simulink model "test_1"  (R2021a)
settings: Solver=ode8  StartTime=0.0  StopTime=6  FixedStep=ts  RelTol=1e-3
undefined symbols (not defined in the file or in its folder): Acid, Lead, ts
libraries: spsDiodeLib x14, spsMosfetLib x12, spsSeriesRLCBranchLib x10, spsCurrentMeasurementLib x8, simulink x7, spsBatteryLib x6, pid_lib x6, spsParallelRLCBranchLib x5, spsMeanLib x3, spsPWMGeneratorDCDCLib x2, spsOnDelayLib x2, spsVoltageMeasurementLib x2
settings Model: Creator=Aditya  LastModifiedBy=Aditya

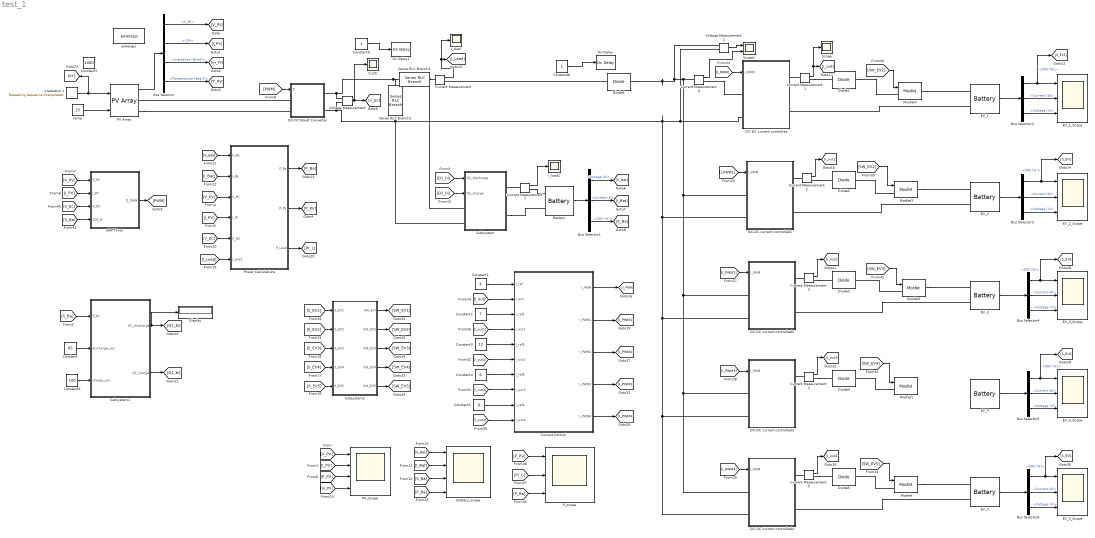
== system test_1 ==
  Battery : spsBatteryLib/Battery  BatType=Lead-Acid  ShowTempParam=off  ThermalPreset=no  ShowAgeParam=off  NomV=60  NomQ=150  SOC=65.01  Batt_Tr=0.1  PresetModel=on  MaxQ=156.25  MinV=45  FullV=65.3289  Dis_rate=30  R=0.004  Normal_OP=46.5417  expZone="[61.0855          0.5]"  current=[6.5 13 32.5]  Units=Time  Tci=20  NomT=20  T2=-30  MaxQ2=4.8  FullV2=7.1  Normal_OP2=5.655  expZone2="[6.58           1]"  Rca=0.6  ti=2000  Dp=0  Neq0=0  Tsim=1e6  Ta1=25  Qeol=5.4*0.9  Reol=0.013333*1.2  Char_age=[2.3478, 3]  Dis_age=[2.3478, 10]  N1=1500  N2=10500  N3=1000  N4=1400  Ta2=45  N5=950
  "Battery_scope " : Scope  NumInputPorts=4
  Bus Selector : BusSelector  OutputSignals=V_PV,I_PV,Irradiance (W/m2),Temperature (deg C)
  Bus Selector1 : BusSelector  OutputSignals=Voltage (V),Current (A),SOC (%)
  Bus Selector{2..6} (5 alike) : BusSelector  OutputSignals=SOC (%),Current (A),Voltage (V)
  Constant : Constant  Value=65
  Constant1 : Constant  Value=4
  Constant2 : Constant  Value=7
  Constant3 : Constant  Value=12
  Constant4 : Constant  Value=6
  Constant5 : Constant  Value=9
  Constant6 : Constant  Value=100
  Constant7 : Constant  Value=1000
  Constant8 : Constant
  Constant9 : Constant
  Current Control : Subsystem
  Current Measurement{,1..7} (8 alike) : spsCurrentMeasurementLib/Current Measurement  PhasorSimulation=off  OutputType=Complex  PSBequivalent=0
  DC-DC Boost Converter : Subsystem
  DC-DC current controlled : Subsystem
  DC-DC current controlled1 : Subsystem
  DC-DC current controlled2 : Subsystem
  DC-DC current controlled3 : Subsystem
  DC-DC current controlled4 : Subsystem
  Diode{1..6} (6 alike) : spsDiodeLib/Diode  Ron=0.001  Lon=0  Vf=0.8  IC=0  UseSnubber=0  Rs=500  Cs=250e-9  Measurements=off
  Display : Display
  EV_1 : spsBatteryLib/Battery  BatType=Lead-Acid  ShowTempParam=off  ThermalPreset=no  ShowAgeParam=off  NomV=48  NomQ=20  SOC=99.7  Batt_Tr=0.1  PresetModel=on  MaxQ=20.8333  MinV=36  FullV=52.2632  Dis_rate=4  R=0.024  Normal_OP=6.2056  expZone="[48.8684    0.0666667]"  current=[6.5 13 32.5]  Units=Time  Tci=20  NomT=20  T2=-30  MaxQ2=4.8  FullV2=7.1  Normal_OP2=5.655  expZone2="[6.58           1]"  Rca=0.6  ti=2000  Dp=0  Neq0=0  Tsim=1e6  Ta1=25  Qeol=5.4*0.9  Reol=0.013333*1.2  Char_age=[2.3478, 3]  Dis_age=[2.3478, 10]  N1=1500  N2=10500  N3=1000  N4=1400  Ta2=45  N5=950
  EV_1_Scope : Scope  NumInputPorts=3
  EV_2 : spsBatteryLib/Battery  BatType=Lead-Acid  ShowTempParam=off  ThermalPreset=no  ShowAgeParam=off  NomV=48  NomQ=30  SOC=99.8  Batt_Tr=0.1  PresetModel=on  MaxQ=31.25  MinV=36  FullV=52.2632  Dis_rate=6  R=0.016  Normal_OP=9.3083  expZone="[48.8684          0.1]"  current=[6.5 13 32.5]  Units=Time  Tci=20  NomT=20  T2=-30  MaxQ2=4.8  FullV2=7.1  Normal_OP2=5.655  expZone2="[6.58           1]"  Rca=0.6  ti=2000  Dp=0  Neq0=0  Tsim=1e6  Ta1=25  Qeol=5.4*0.9  Reol=0.013333*1.2  Char_age=[2.3478, 3]  Dis_age=[2.3478, 10]  N1=1500  N2=10500  N3=1000  N4=1400  Ta2=45  N5=950
  EV_2_Scope : Scope  NumInputPorts=3
  EV_3 : spsBatteryLib/Battery  BatType=Lead-Acid  ShowTempParam=off  ThermalPreset=no  ShowAgeParam=off  NomV=48  NomQ=50  SOC=99.9  Batt_Tr=0.1  PresetModel=on  MaxQ=52.0833  MinV=36  FullV=52.2632  Dis_rate=10  R=0.0096  Normal_OP=15.5139  expZone="[48.8684     0.166667]"  current=[6.5 13 32.5]  Units=Time  Tci=20  NomT=20  T2=-30  MaxQ2=4.8  FullV2=7.1  Normal_OP2=5.655  expZone2="[6.58           1]"  Rca=0.6  ti=2000  Dp=0  Neq0=0  Tsim=1e6  Ta1=25  Qeol=5.4*0.9  Reol=0.013333*1.2  Char_age=[2.3478, 3]  Dis_age=[2.3478, 10]  N1=1500  N2=10500  N3=1000  N4=1400  Ta2=45  N5=950
  EV_3_Scope : Scope  NumInputPorts=3
  EV_4 : spsBatteryLib/Battery  BatType=Lead-Acid  ShowTempParam=off  ThermalPreset=no  ShowAgeParam=off  NomV=48  NomQ=28  SOC=99.95  Batt_Tr=0.1  PresetModel=on  MaxQ=29.1667  MinV=36  FullV=52.2632  Dis_rate=5.6  R=0.017143  Normal_OP=8.6878  expZone="[48.8684    0.0933333]"  current=[6.5 13 32.5]  Units=Time  Tci=20  NomT=20  T2=-30  MaxQ2=4.8  FullV2=7.1  Normal_OP2=5.655  expZone2="[6.58           1]"  Rca=0.6  ti=2000  Dp=0  Neq0=0  Tsim=1e6  Ta1=25  Qeol=5.4*0.9  Reol=0.013333*1.2  Char_age=[2.3478, 3]  Dis_age=[2.3478, 10]  N1=1500  N2=10500  N3=1000  N4=1400  Ta2=45  N5=950
  EV_4_Scope : Scope  NumInputPorts=3
  EV_5 : spsBatteryLib/Battery  BatType=Lead-Acid  ShowTempParam=off  ThermalPreset=no  ShowAgeParam=off  NomV=48  NomQ=40  SOC=99.5  Batt_Tr=0.1  PresetModel=on  MaxQ=41.6667  MinV=36  FullV=52.2632  Dis_rate=8  R=0.012  Normal_OP=12.4111  expZone="[48.8684     0.133333]"  current=[6.5 13 32.5]  Units=Time  Tci=20  NomT=20  T2=-30  MaxQ2=4.8  FullV2=7.1  Normal_OP2=5.655  expZone2="[6.58           1]"  Rca=0.6  ti=2000  Dp=0  Neq0=0  Tsim=1e6  Ta1=25  Qeol=5.4*0.9  Reol=0.013333*1.2  Char_age=[2.3478, 3]  Dis_age=[2.3478, 10]  N1=1500  N2=10500  N3=1000  N4=1400  Ta2=45  N5=950
  EV_5_Scope : Scope  NumInputPorts=3
  I_load : Scope
  I_load1 : Scope
  MPPT PnO : Subsystem
  Mosfet{,1..4} (5 alike) : spsMosfetLib/Mosfet  Ron=0.1  Lon=0  Rd=0.01  Vfd=0  IC=0  Rs=1e5  Cs=inf  Measurements=off
  On Delay : spsOnDelayLib/On Delay  DelayType=On delay  delay=1.25  ic=0  Ts=0
      settings: SourceProductBaseCode=PS
  On Delay1 : spsOnDelayLib/On Delay  DelayType=On delay  delay=0.05  ic=0  Ts=0
      settings: SourceProductBaseCode=PS
  PV Array : spsPVArrayLib/PV Array  Npar=4  Nser=4  PlotType=one module @ 25 deg.C & specified irradiances  S_vec="[ 1000 800 500  250 ]"  Temp_C_vec="[0 25 50  ]"  ModuleName=User-defined  PlotWhenSelected=on  Pm=204.7968  Ncell=60  Voc=22.46  Isc=11.65  Vm=18.72  Im=10.94  beta_Voc_pc=-0.3609  alpha_Isc_pc=0.102  beta_Voc=-0.081058  alpha_Isc=0.011883  IL=11.6575  I0=4.2837e-10  nI=0.60677  Rsh=131.4101  Rs=0.084786  RobustModel=off  RobustCellTemperature=25  BAL=on  Tc=Tc  Tfilter=5e-5
  PV_Scope : Scope  NumInputPorts=4
  P_scope : Scope  NumInputPorts=3
  Power Calculations : Subsystem
  Scope : Scope
  Scope1 : Scope  NumInputPorts=2
  Series RLC Branch2 : spsSeriesRLCBranchLib/Series RLC Branch  LConnTagsString=__new0  RConnTagsString=__new0  BranchType=C  Resistance=1.2  Inductance=1e-3  SetiL0=off  InitialCurrent=0  Capacitance=15000e-6  Setx0=on  InitialVoltage=60  Measurements=None
  Series RLC Branch3 : spsSeriesRLCBranchLib/Series RLC Branch  LConnTagsString=__new0  RConnTagsString=__new0  BranchType=L  Resistance=1.2  Inductance=0.325e-3  SetiL0=off  InitialCurrent=0  Capacitance=15000e-6  Setx0=on  InitialVoltage=70  Measurements=None
  Subsystem : Subsystem
  Subsystem1 : Subsystem
  Subsystem2 : Subsystem
  V_DC : Scope
  Voltage Measurement : spsVoltageMeasurementLib/Voltage Measurement  PhasorSimulation=off  OutputType=Complex  PSBequivalent=0
  Voltage Measurement2 : spsVoltageMeasurementLib/Voltage Measurement  PhasorSimulation=off  OutputType=Complex  PSBequivalent=0
  irradiation 1 : simulink/Sources/Repeating Sequence Interpolated  OutValues=[0 0 0 0 0 100 200 300 400 700 800 900 1000 975 900 800 700 400 300 200 0 0 0 0].'  TimeValues=[0 0.25 0.50 0.75 1 1.25 1.50 1.75 2 2.25 2.75 3 3.25 3.50 3.75 4 4.25 4.5 4.75 5 5.25 5.5 5.75 6 ].'  LookUpMeth=Interpolation-Use End Values  tsamp=0.1  OutMin=[]  OutMax=[]  OutDataTypeStr=double  OutputDataTypeScalingMode=double  OutDataType=fixdt(0,8)  OutScaling=2^-10
  powergui : spspowerguiLib/powergui  Priority=1  SimulationMode=Discrete  SampleTime=ts  frequency=60  Iterations=50  frequencyindice=0  Pbase=100e6  ErrMax=1e-4  UnitsV=kV  UnitsW=MW  buscounter=0  FunctionMessages=off  echomessages=off  EnableUseOfTLC=off  CurrentSourceSwitches=off  DisableSnubberDevices=off  DisableRonSwitches=off  DisableVfSwitches=off  DisplayEquations=off  AutomaticDiscreteSolvers=off  SolverType=Tustin/Backward Euler (TBE)  Interpol=off  ExternalGateDelay=off  methode=off  Ts=100  x0status=blocks  SPID=on  SwTol=0  HookPort=off  NonlinearTolerance=1e-4  nMaxIteration=100  ContinueOnMaxIteration=off  RestoreLinks=warning  ResistiveCurrentMeasurement=off  Frange=[0:2:500]  Ylog=off  Xlog=on  ShowGrid=off  save=on  variable=ZData  structure=V_BATT  ZoomFFT=on  StartTime=0.604  cycles=7  DisplayStyle=1  fundamental=50  FreqAxis=off  MaxFrequency=200  frequencyindicesteady=1  RmsSteady=1  display=off
  temp : Constant  Value=25
  wires:
  Current Control/2(I_PWM1) -> [I_PWM1]
  Constant2/1 -> Current Control/3(I_ref1)
  [V_PV] -> Power Calculations/3(V_PV)
  Power Calculations/1(P_Ba) -> [P_Ba]
  Current Measurement2/1 -> [I_out1]
  Bus Selector3/2 -> EV_2_Scope/2  "<Current (A)>"
  [V_DC] -> Power Calculations/5(V_DC)
  [I_out1] -> Current Control/4(I_out1)
  EV_2/1 -> Bus Selector3/1
  Constant1/1 -> Current Control/1(I_ref)
  [PWM] -> DC-DC Boost Converter/1(D)
  irradiation 1/1 -> PV Array/1, [irr]
  [I_PWM1] -> DC-DC current controlled1/1(I_PWM)
  Bus Selector3/1 -> [S_EV2], EV_2_Scope/1  "<SOC (%)>"
  Battery/1 -> Bus Selector1/1
  Bus Selector/1 -> [V_PV]  "<V_PV>"
  Current Control/1(I_PWM) -> [I_PWM]
  EV_1/1 -> Bus Selector2/1
  Bus Selector3/3 -> EV_2_Scope/3  "<Voltage (V)>"
  [I_PV] -> Power Calculations/4(I_PV)
  Bus Selector2/2 -> EV_1_Scope/2  "<Current (A)>"
  Power Calculations/3(P_Load) -> [Pr_L]
  [I_Bat] -> "Battery_scope "/2
  [V_Bat] -> "Battery_scope "/1
  Bus Selector2/3 -> EV_1_Scope/3  "<Voltage (V)>"
  [I_Load] -> Power Calculations/6(I_Load)
  [I_PWM] -> DC-DC current controlled/1(I_PWM)
  [I_out] -> Current Control/2(I_out)
  [V_Bat] -> Power Calculations/1(V_Ba)
  Power Calculations/2(P_PV) -> [P_PV]
  Current Measurement/1 -> I_load/1, [I_Load]
  Current Measurement1/1 -> Scope/1, [I_out]
  [V_PV] -> PV_Scope/1
  [P_PV] -> P_scope/1
  Bus Selector1/2 -> [I_Bat]  "<Current (A)>"
  [P_PV] -> PV_Scope/3
  [P_Ba] -> P_scope/3
  [Irr_PV] -> PV_Scope/4
  [I_PV] -> PV_Scope/2
  [P_Ba] -> "Battery_scope "/4
  Bus Selector1/3 -> [S_Ba]  "<SOC (%)>"
  [S_Ba] -> "Battery_scope "/3
  [I_Bat] -> Power Calculations/2(I_Ba)
  [V_DC] -> MPPT PnO/3(V_DC)
  Bus Selector1/1 -> [V_Bat]  "<Voltage (V)>"
  [V_PV] -> MPPT PnO/1(V_PV)
  [S_Ba] -> MPPT PnO/4(SOC_B)
  MPPT PnO/1(D_PWM) -> [PWM]
  [I_PV] -> MPPT PnO/2(I_PV)
  Bus Selector2/1 -> [S_EV1], EV_1_Scope/1  "<SOC (%)>"
  temp/1 -> PV Array/2
  Bus Selector/2 -> [I_PV]  "<I_PV>"
  PV Array/1 -> Bus Selector/1
  [Pr_L] -> P_scope/2
  Bus Selector/4 -> [T_PV]  "<Temperature (deg C)>"
  Bus Selector/3 -> [Irr_PV]  "<Irradiance (W/m2)>"
  Bus Selector4/3 -> EV_3_Scope/3  "<Voltage (V)>"
  Bus Selector4/1 -> [S_EV3], EV_3_Scope/1  "<SOC (%)>"
  [I_PWM2] -> DC-DC current controlled2/1(I_PWM)
  EV_3/1 -> Bus Selector4/1
  Bus Selector4/2 -> EV_3_Scope/2  "<Current (A)>"
  Current Measurement3/1 -> [I_out2]
  Current Measurement4/1 -> [I_out3]
  Bus Selector5/2 -> EV_4_Scope/2  "<Current (A)>"
  EV_4/1 -> Bus Selector5/1
  [I_PWM3] -> DC-DC current controlled3/1(I_PWM)
  Bus Selector5/1 -> [S_EV4], EV_4_Scope/1  "<SOC (%)>"
  Bus Selector5/3 -> EV_4_Scope/3  "<Voltage (V)>"
  Bus Selector6/3 -> EV_5_Scope/3  "<Voltage (V)>"
  Bus Selector6/1 -> [S_EV5], EV_5_Scope/1  "<SOC (%)>"
  [I_PWM4] -> DC-DC current controlled4/1(I_PWM)
  EV_5/1 -> Bus Selector6/1
  Bus Selector6/2 -> EV_5_Scope/2  "<Current (A)>"
  Current Measurement5/1 -> [I_out4]
  [I_out4] -> Current Control/10(I_out4)
  [I_out3] -> Current Control/8(I_out3)
  Current Control/4(I_PWM3) -> [I_PWM3]
  Current Control/5(I_PWM4) -> [I_PWM4]
  [I_out2] -> Current Control/6(I_out2)
  Current Control/3(I_PWM2) -> [I_PWM2]
  Constant5/1 -> Current Control/9(I_ref4)
  Constant4/1 -> Current Control/7(I_ref3)
  Constant3/1 -> Current Control/5(I_ref2)
  Voltage Measurement2/1 -> Scope1/1
  Subsystem1/1(Q1_discharge) -> Display/1, [Q1_bi]
  Subsystem1/2(Q2_charge) -> [Q2_bi]
  [S_Ba] -> Subsystem1/1(S_bt)
  Constant/1 -> Subsystem1/2(discharge_soc)
  Constant6/1 -> Subsystem1/3(charge_soc)
  [Q2_bi] -> Subsystem/2(Q2_charge)
  [Q1_bi] -> Subsystem/1(Q1_discharge)
  [S_EV1] -> Subsystem2/1(S_EV1)
  [S_EV4] -> Subsystem2/4(S_EV4)
  [S_EV5] -> Subsystem2/5(S_EV5)
  [S_EV2] -> Subsystem2/2(S_EV2)
  [S_EV3] -> Subsystem2/3(S_EV3)
  Subsystem2/1(SW_EV!) -> [SW_EV1]
  Subsystem2/2(SW_EV2) -> [SW_EV2]
  Subsystem2/3(SW_EV3) -> [SW_EV3]
  Subsystem2/4(SW_EV4) -> [SW_EV4]
  Subsystem2/5(SW_EV5) -> [SW_EV5]
  [SW_EV1] -> Mosfet4/1
  [SW_EV2] -> Mosfet3/1
  [SW_EV3] -> Mosfet2/1
  [SW_EV4] -> Mosfet1/1
  [SW_EV5] -> Mosfet/1
  Current Measurement7/1 -> I_load1/1
  Constant8/1 -> On Delay/1
  Current Measurement6/1 -> Scope1/2
  Constant9/1 -> On Delay1/1
  Voltage Measurement/1 -> V_DC/1, [V_DC]
  connections:
  Current Measurement2/RConn1 -- Diode2/LConn1
  Current Measurement1/LConn1 -- DC-DC current controlled/RConn1
  Current Measurement1/RConn1 -- Diode1/LConn1
  DC-DC Boost Converter/LConn1 -- PV Array/RConn1
  PV Array/RConn2 -- DC-DC Boost Converter/LConn2
  Current Measurement2/LConn1 -- DC-DC current controlled1/RConn1
  Current Measurement3/LConn1 -- DC-DC current controlled2/RConn1
  Current Measurement3/RConn1 -- Diode3/LConn1
  Current Measurement4/LConn1 -- DC-DC current controlled3/RConn1
  Current Measurement4/RConn1 -- Diode4/LConn1
  Current Measurement5/LConn1 -- DC-DC current controlled4/RConn1
  Current Measurement5/RConn1 -- Diode5/LConn1
  Current Measurement/LConn1 -- Series RLC Branch3/LConn1 -- Subsystem/LConn1
  Diode6/RConn1 -- Voltage Measurement2/LConn1 -- DC-DC current controlled4/LConn1 -- DC-DC current controlled3/LConn1 -- DC-DC current controlled2/LConn1 -- DC-DC current controlled1/LConn1 -- Current Measurement6/LConn1
  Subsystem/RConn2 -- Battery/LConn2
  Diode1/RConn1 -- Mosfet4/LConn1
  Mosfet3/LConn1 -- Diode2/RConn1
  Mosfet2/LConn1 -- Diode3/RConn1
  Mosfet1/LConn1 -- Diode4/RConn1
  Mosfet/LConn1 -- Diode5/RConn1
  Current Measurement7/LConn1 -- Subsystem/RConn1
  Current Measurement7/RConn1 -- Battery/LConn1
  Current Measurement6/RConn1 -- DC-DC current controlled/LConn1
  Mosfet2/RConn1 -- EV_3/LConn1
  DC-DC current controlled2/LConn2 -- DC-DC current controlled4/LConn2 -- DC-DC current controlled3/LConn2 -- DC-DC current controlled1/LConn2 -- Subsystem/LConn2 -- Voltage Measurement/LConn2 -- DC-DC Boost Converter/RConn2 -- Series RLC Branch2/RConn1 -- DC-DC current controlled/LConn2 -- Voltage Measurement2/LConn2
  Diode6/LConn1 -- Current Measurement/RConn1
  Series RLC Branch3/RConn1 -- Voltage Measurement/LConn1 -- DC-DC Boost Converter/RConn1 -- Series RLC Branch2/LConn1
  Mosfet4/RConn1 -- EV_1/LConn1
  EV_1/LConn2 -- DC-DC current controlled/RConn2
  Mosfet3/RConn1 -- EV_2/LConn1
  EV_2/LConn2 -- DC-DC current controlled1/RConn2
  EV_3/LConn2 -- DC-DC current controlled2/RConn2
  Mosfet/RConn1 -- EV_5/LConn1
  EV_5/LConn2 -- DC-DC current controlled4/RConn2

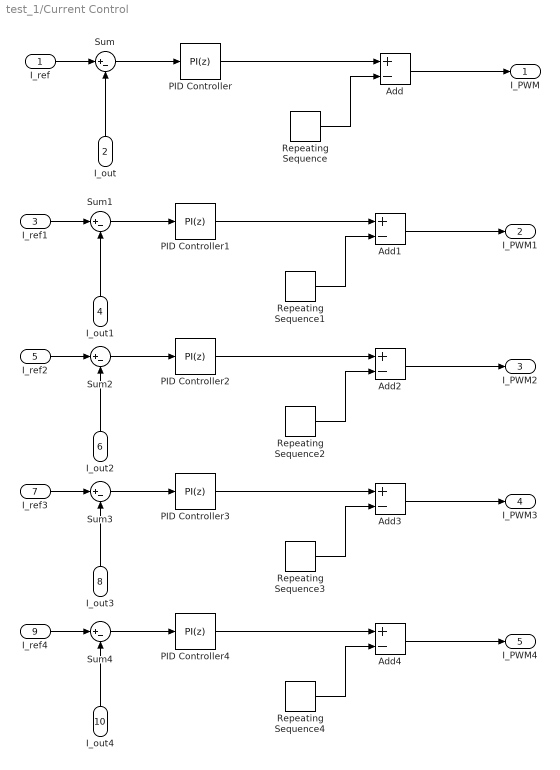
== system test_1/Current Control ==
  I_ref : Inport
  I_out : Inport  Port=2
  I_ref1 : Inport  Port=3
  I_out1 : Inport  Port=4
  I_ref2 : Inport  Port=5
  I_out2 : Inport  Port=6
  I_ref3 : Inport  Port=7
  I_out3 : Inport  Port=8
  I_ref4 : Inport  Port=9
  I_out4 : Inport  Port=10
  Add{,1..4} (5 alike) : Sum  Inputs=+-
  PID Controller{,1..4} (5 alike) : pid_lib/PID Controller  Controller=PI  Form=Parallel  TimeDomain=Discrete-time  UseExternalTs=off  SampleTime=-1  IntegratorMethod=Forward Euler  FilterMethod=Forward Euler  ControllerParametersSource=internal  P=0.4928  I=0.93  D=0  UseFilter=on  N=100  TunerSelectOption=Transfer Function Based (PID Tuner App)  InitialConditionSource=internal  InitialConditionForIntegrator=0  InitialConditionForFilter=0  DifferentiatorICPrevScaledInput=0  ExternalReset=none  TrackingMode=off  Kt=1  LimitOutput=off  SatLimitsSource=internal  UpperSaturationLimit=inf  LowerSaturationLimit=-inf  LinearizeAsGain=on  AntiWindupMode=none  Kb=1  POutMin=[]  POutMax=[]  IOutMin=[]  IOutMax=[]  DOutMin=[]  DOutMax=[]  NOutMin=[]  NOutMax=[]  SumOutMin=[]  SumOutMax=[]  SaturationOutMin=[]  SaturationOutMax=[]  PParamMin=[]  PParamMax=[]  IParamMin=[]  IParamMax=[]  DParamMin=[]  DParamMax=[]  NParamMin=[]  NParamMax=[]  KbParamMin=[]  KbParamMax=[]  KtParamMin=[]  KtParamMax=[]  KbOutMin=[]  KbOutMax=[]  KtOutMin=[]  KtOutMax=[]  IntegratorOutMin=[]  IntegratorOutMax=[]  FilterOutMin=[]  FilterOutMax=[]  SumI1OutMin=[]  SumI1OutMax=[]  SumI2OutMin=[]  SumI2OutMax=[]  SumI3OutMin=[]  SumI3OutMax=[]  SumI4OutMin=[]  SumI4OutMax=[]  SumDOutMin=[]  SumDOutMax=[]  DifferentiatorOutMin=[]  DifferentiatorOutMax=[]  FilterDiffOutCoefMin=[]  FilterDiffOutCoefMax=[]  ReciprocalOutMin=[]  ReciprocalOutMax=[]  SumDenOutMin=[]  SumDenOutMax=[]  SumNumOutMin=[]  SumNumOutMax=[]  DivideOutMin=[]  DivideOutMax=[]  UdiffTsProdOutMin=[]  UdiffTsProdOutMax=[]  NTsProdOutMin=[]  NTsProdOutMax=[]  UintegralTsProdOutMin=[]  UintegralTsProdOutMax=[]  UngainTsProdOutMin=[]  UngainTsProdOutMax=[]  IntegratorContinuousStateAttributes=''  IntegratorStateMustResolveToSignalObject=off  IntegratorRTWStateStorageClass=Auto  FilterContinuousStateAttributes=''  FilterStateMustResolveToSignalObject=off  FilterRTWStateStorageClass=Auto  ParallelPVariant=InternalParameters  IdealPVariant=Disabled  IVariant=InternalParameters  DVariant=Disabled  IntegratorVariant=Discrete  SatVariant=Disabled  AWVariant=Passthrough  PCopyVariant=Disabled  TRVariant=Disabled  FdbkBlocksVariant=Forward  IdealPFdbkVariant=Disabled  SatFdbkVariant=Disabled  DerivativeFilterVariant=Disabled  NVariant=Disabled  NCopyVariant=Disabled_SignalSpec  FilterICVariant=Disabled  IntegratorICVariant=InternalICs  ExternalResetVariant=Disabled  TRSumVariant=Passthrough  SumFdbkVariant=Disabled  SumVariant=Sum_PI  TsampFilterVariant=InternalTs  TsampNgainVariant=Passthrough  TsampIntegralVariant=Passthrough  ExternalSaturationOutDataTypeStr=Inherit: Same as second input
  Repeating Sequence{,1..4} (5 alike) : simulink/Sources/Repeating Sequence  rep_seq_t=[0 0.25/5000 0.5/5000 0.75/5000 1/5000]  rep_seq_y=[0 -1 0 1 0]
  Sum{,1..4} (5 alike) : Sum  Inputs=|+-
  I_PWM : Outport
  I_PWM1 : Outport  Port=2
  I_PWM2 : Outport  Port=3
  I_PWM3 : Outport  Port=4
  I_PWM4 : Outport  Port=5
  wires:
  Sum/1 -> PID Controller/1
  PID Controller/1 -> Add/1
  Repeating Sequence/1 -> Add/2
  I_out/1 -> Sum/2
  Add/1 -> I_PWM/1
  I_ref/1 -> Sum/1
  I_ref1/1 -> Sum1/1
  Add1/1 -> I_PWM1/1
  I_out1/1 -> Sum1/2
  Repeating Sequence1/1 -> Add1/2
  PID Controller1/1 -> Add1/1
  Sum1/1 -> PID Controller1/1
  Sum2/1 -> PID Controller2/1
  PID Controller2/1 -> Add2/1
  Repeating Sequence2/1 -> Add2/2
  I_out2/1 -> Sum2/2
  Add2/1 -> I_PWM2/1
  I_ref2/1 -> Sum2/1
  I_ref3/1 -> Sum3/1
  Add3/1 -> I_PWM3/1
  I_out3/1 -> Sum3/2
  Repeating Sequence3/1 -> Add3/2
  PID Controller3/1 -> Add3/1
  Sum3/1 -> PID Controller3/1
  Sum4/1 -> PID Controller4/1
  PID Controller4/1 -> Add4/1
  Repeating Sequence4/1 -> Add4/2
  I_out4/1 -> Sum4/2
  Add4/1 -> I_PWM4/1
  I_ref4/1 -> Sum4/1

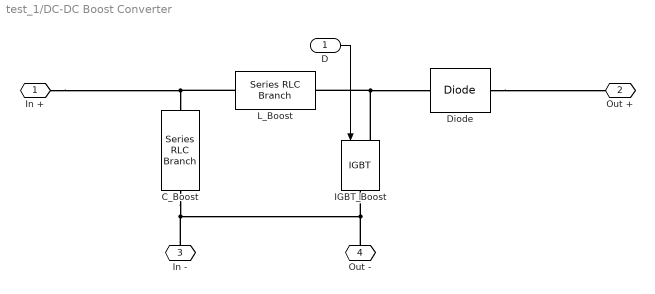
== system test_1/DC-DC Boost Converter ==
  D : Inport
  C_Boost : spsSeriesRLCBranchLib/Series RLC Branch  LConnTagsString=__new0  RConnTagsString=__new0  BranchType=C  Resistance=0.01  Inductance=1e-3  SetiL0=off  InitialCurrent=0  Capacitance=2200e-6  Setx0=off  InitialVoltage=0  Measurements=None
  Diode : spsDiodeLib/Diode  Ron=0.001  Lon=0  Vf=0.8  IC=0  UseSnubber=0  Rs=500  Cs=250e-9  Measurements=off
  IGBT_Boost : spsIGBTLib/IGBT  Ron=0.001  Lon=0  Vf=0  Tf=0  Tt=0  IC=0  Rs=1e5  Cs=inf  Measurements=off
  L_Boost : spsSeriesRLCBranchLib/Series RLC Branch  LConnTagsString=__new0  RConnTagsString=__new0  BranchType=RL  Resistance=0.05  Inductance=0.325e-3  SetiL0=off  InitialCurrent=0  Capacitance=1e-6  Setx0=off  InitialVoltage=0  Measurements=None
  In + : PMIOPort  Side=Left
  Out + : PMIOPort  Port=2  Side=Right
  In - : PMIOPort  Port=3  Side=Left
  Out - : PMIOPort  Port=4  Side=Right
  wires:
  D/1 -> IGBT_Boost/1
  connections:
  IGBT_Boost/LConn1 -- Diode/LConn1 -- L_Boost/RConn1
  Diode/RConn1 -- Out +/RConn1
  L_Boost/LConn1 -- In +/RConn1 -- C_Boost/LConn1
  C_Boost/RConn1 -- In -/RConn1 -- Out -/RConn1 -- IGBT_Boost/RConn1

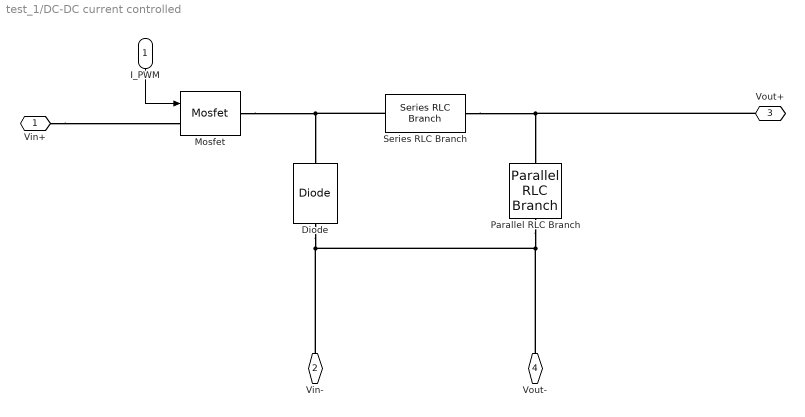
== system test_1/DC-DC current controlled ==
  I_PWM : Inport
  Diode : spsDiodeLib/Diode  Ron=0.001  Lon=0  Vf=0.8  IC=0  UseSnubber=0  Rs=500  Cs=250e-9  Measurements=off
  Mosfet : spsMosfetLib/Mosfet  Ron=0.1  Lon=0  Rd=0.01  Vfd=0  IC=0  Rs=1e5  Cs=inf  Measurements=off
  Parallel RLC Branch : spsParallelRLCBranchLib/Parallel RLC Branch  LConnTagsString=a  RConnTagsString=__new0  BranchType=C  Resistance=1  Inductance=1e-3  SetiL0=off  InitialCurrent=0  Capacitance=200e-6  Setx0=off  InitialVoltage=0  Measurements=None
  Series RLC Branch : spsSeriesRLCBranchLib/Series RLC Branch  LConnTagsString=__new0  RConnTagsString=__new0  BranchType=L  Resistance=10  Inductance=100e-3  SetiL0=off  InitialCurrent=0  Capacitance=1e-6  Setx0=off  InitialVoltage=0  Measurements=None
  Vin+ : PMIOPort  Side=Left
  Vin- : PMIOPort  Port=2  Side=Left
  Vout+ : PMIOPort  Port=3  Side=Right
  Vout- : PMIOPort  Port=4  Side=Right
  wires:
  I_PWM/1 -> Mosfet/1
  connections:
  Mosfet/RConn1 -- Diode/RConn1 -- Series RLC Branch/LConn1
  Vin-/RConn1 -- Vout-/RConn1 -- Parallel RLC Branch/RConn1 -- Diode/LConn1
  Vout+/RConn1 -- Series RLC Branch/RConn1 -- Parallel RLC Branch/LConn1
  Vin+/RConn1 -- Mosfet/LConn1

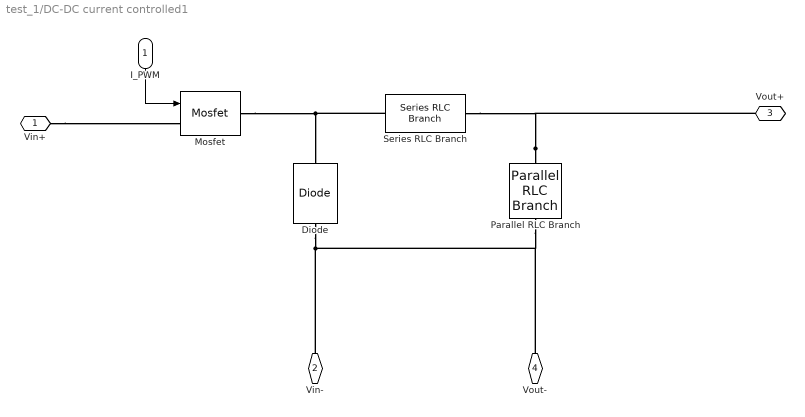
== system test_1/DC-DC current controlled1 ==
  I_PWM : Inport
  Diode : spsDiodeLib/Diode  Ron=0.001  Lon=0  Vf=0.8  IC=0  UseSnubber=0  Rs=500  Cs=250e-9  Measurements=off
  Mosfet : spsMosfetLib/Mosfet  Ron=0.1  Lon=0  Rd=0.01  Vfd=0  IC=0  Rs=1e5  Cs=inf  Measurements=off
  Parallel RLC Branch : spsParallelRLCBranchLib/Parallel RLC Branch  LConnTagsString=a  RConnTagsString=__new0  BranchType=C  Resistance=1  Inductance=1e-3  SetiL0=off  InitialCurrent=0  Capacitance=200e-6  Setx0=off  InitialVoltage=0  Measurements=None
  Series RLC Branch : spsSeriesRLCBranchLib/Series RLC Branch  LConnTagsString=__new0  RConnTagsString=__new0  BranchType=L  Resistance=10  Inductance=100e-3  SetiL0=off  InitialCurrent=0  Capacitance=1e-6  Setx0=off  InitialVoltage=0  Measurements=None
  Vin+ : PMIOPort  Side=Left
  Vin- : PMIOPort  Port=2  Side=Left
  Vout+ : PMIOPort  Port=3  Side=Right
  Vout- : PMIOPort  Port=4  Side=Right
  wires:
  I_PWM/1 -> Mosfet/1
  connections:
  Vin+/RConn1 -- Mosfet/LConn1
  Parallel RLC Branch/LConn1 -- Series RLC Branch/RConn1 -- Vout+/RConn1
  Diode/LConn1 -- Parallel RLC Branch/RConn1 -- Vout-/RConn1 -- Vin-/RConn1
  Series RLC Branch/LConn1 -- Diode/RConn1 -- Mosfet/RConn1

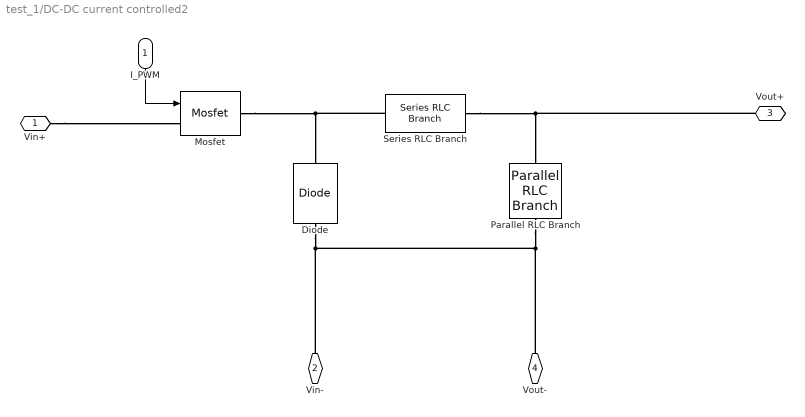
== system test_1/DC-DC current controlled2 ==
  I_PWM : Inport
  Diode : spsDiodeLib/Diode  Ron=0.001  Lon=0  Vf=0.8  IC=0  UseSnubber=0  Rs=500  Cs=250e-9  Measurements=off
  Mosfet : spsMosfetLib/Mosfet  Ron=0.1  Lon=0  Rd=0.01  Vfd=0  IC=0  Rs=1e5  Cs=inf  Measurements=off
  Parallel RLC Branch : spsParallelRLCBranchLib/Parallel RLC Branch  LConnTagsString=a  RConnTagsString=__new0  BranchType=C  Resistance=1  Inductance=1e-3  SetiL0=off  InitialCurrent=0  Capacitance=200e-6  Setx0=off  InitialVoltage=0  Measurements=None
  Series RLC Branch : spsSeriesRLCBranchLib/Series RLC Branch  LConnTagsString=__new0  RConnTagsString=__new0  BranchType=L  Resistance=10  Inductance=100e-3  SetiL0=off  InitialCurrent=0  Capacitance=1e-6  Setx0=off  InitialVoltage=0  Measurements=None
  Vin+ : PMIOPort  Side=Left
  Vin- : PMIOPort  Port=2  Side=Left
  Vout+ : PMIOPort  Port=3  Side=Right
  Vout- : PMIOPort  Port=4  Side=Right
  wires:
  I_PWM/1 -> Mosfet/1
  connections:
  Mosfet/RConn1 -- Diode/RConn1 -- Series RLC Branch/LConn1
  Vin-/RConn1 -- Vout-/RConn1 -- Parallel RLC Branch/RConn1 -- Diode/LConn1
  Vout+/RConn1 -- Series RLC Branch/RConn1 -- Parallel RLC Branch/LConn1
  Vin+/RConn1 -- Mosfet/LConn1

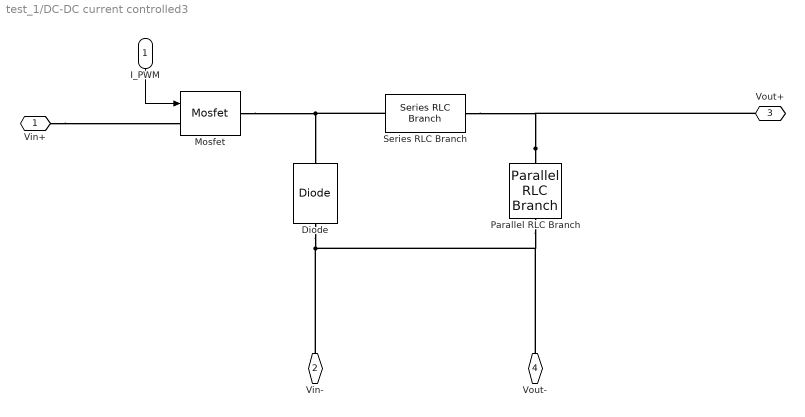
== system test_1/DC-DC current controlled3 ==
  I_PWM : Inport
  Diode : spsDiodeLib/Diode  Ron=0.001  Lon=0  Vf=0.8  IC=0  UseSnubber=0  Rs=500  Cs=250e-9  Measurements=off
  Mosfet : spsMosfetLib/Mosfet  Ron=0.1  Lon=0  Rd=0.01  Vfd=0  IC=0  Rs=1e5  Cs=inf  Measurements=off
  Parallel RLC Branch : spsParallelRLCBranchLib/Parallel RLC Branch  LConnTagsString=a  RConnTagsString=__new0  BranchType=C  Resistance=1  Inductance=1e-3  SetiL0=off  InitialCurrent=0  Capacitance=200e-6  Setx0=off  InitialVoltage=0  Measurements=None
  Series RLC Branch : spsSeriesRLCBranchLib/Series RLC Branch  LConnTagsString=__new0  RConnTagsString=__new0  BranchType=L  Resistance=10  Inductance=100e-3  SetiL0=off  InitialCurrent=0  Capacitance=1e-6  Setx0=off  InitialVoltage=0  Measurements=None
  Vin+ : PMIOPort  Side=Left
  Vin- : PMIOPort  Port=2  Side=Left
  Vout+ : PMIOPort  Port=3  Side=Right
  Vout- : PMIOPort  Port=4  Side=Right
  wires:
  I_PWM/1 -> Mosfet/1
  connections:
  Vin+/RConn1 -- Mosfet/LConn1
  Parallel RLC Branch/LConn1 -- Series RLC Branch/RConn1 -- Vout+/RConn1
  Diode/LConn1 -- Parallel RLC Branch/RConn1 -- Vout-/RConn1 -- Vin-/RConn1
  Series RLC Branch/LConn1 -- Diode/RConn1 -- Mosfet/RConn1

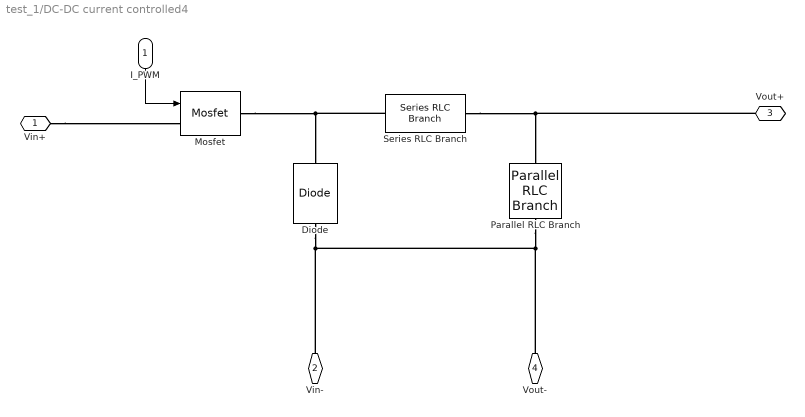
== system test_1/DC-DC current controlled4 ==
  I_PWM : Inport
  Diode : spsDiodeLib/Diode  Ron=0.001  Lon=0  Vf=0.8  IC=0  UseSnubber=0  Rs=500  Cs=250e-9  Measurements=off
  Mosfet : spsMosfetLib/Mosfet  Ron=0.1  Lon=0  Rd=0.01  Vfd=0  IC=0  Rs=1e5  Cs=inf  Measurements=off
  Parallel RLC Branch : spsParallelRLCBranchLib/Parallel RLC Branch  LConnTagsString=a  RConnTagsString=__new0  BranchType=C  Resistance=1  Inductance=1e-3  SetiL0=off  InitialCurrent=0  Capacitance=200e-6  Setx0=off  InitialVoltage=0  Measurements=None
  Series RLC Branch : spsSeriesRLCBranchLib/Series RLC Branch  LConnTagsString=__new0  RConnTagsString=__new0  BranchType=L  Resistance=10  Inductance=100e-3  SetiL0=off  InitialCurrent=0  Capacitance=1e-6  Setx0=off  InitialVoltage=0  Measurements=None
  Vin+ : PMIOPort  Side=Left
  Vin- : PMIOPort  Port=2  Side=Left
  Vout+ : PMIOPort  Port=3  Side=Right
  Vout- : PMIOPort  Port=4  Side=Right
  wires:
  I_PWM/1 -> Mosfet/1
  connections:
  Mosfet/RConn1 -- Diode/RConn1 -- Series RLC Branch/LConn1
  Vin-/RConn1 -- Vout-/RConn1 -- Parallel RLC Branch/RConn1 -- Diode/LConn1
  Vout+/RConn1 -- Series RLC Branch/RConn1 -- Parallel RLC Branch/LConn1
  Vin+/RConn1 -- Mosfet/LConn1

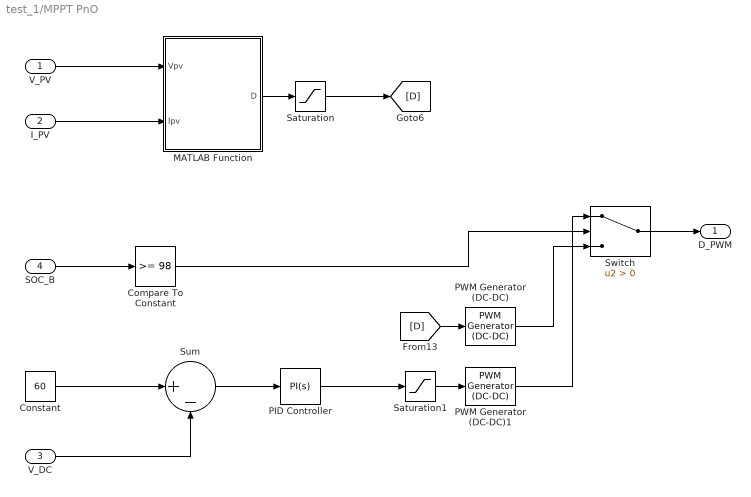
== system test_1/MPPT PnO ==
  V_PV : Inport
  I_PV : Inport  Port=2
  V_DC : Inport  Port=3
  SOC_B : Inport  Port=4
  Compare To Constant : simulink/Logic and Bit Operations/Compare To Constant  relop=>=  const=98  OutDataTypeStr=boolean
  Constant : Constant  Value=60
  MATLAB Function : MATLAB Function  TreatAsAtomicUnit=on
  PID Controller : pid_lib/PID Controller  Controller=PI  Form=Parallel  TimeDomain=Continuous-time  UseExternalTs=off  SampleTime=-1  IntegratorMethod=Forward Euler  FilterMethod=Forward Euler  ControllerParametersSource=internal  P=0.1  I=0.1  D=0  UseFilter=on  N=100  TunerSelectOption=Transfer Function Based (PID Tuner App)  InitialConditionSource=internal  InitialConditionForIntegrator=0  InitialConditionForFilter=0  DifferentiatorICPrevScaledInput=0  ExternalReset=none  TrackingMode=off  Kt=1  LimitOutput=off  SatLimitsSource=internal  UpperSaturationLimit=inf  LowerSaturationLimit=-inf  LinearizeAsGain=on  AntiWindupMode=none  Kb=1  POutMin=[]  POutMax=[]  IOutMin=[]  IOutMax=[]  DOutMin=[]  DOutMax=[]  NOutMin=[]  NOutMax=[]  SumOutMin=[]  SumOutMax=[]  SaturationOutMin=[]  SaturationOutMax=[]  PParamMin=[]  PParamMax=[]  IParamMin=[]  IParamMax=[]  DParamMin=[]  DParamMax=[]  NParamMin=[]  NParamMax=[]  KbParamMin=[]  KbParamMax=[]  KtParamMin=[]  KtParamMax=[]  KbOutMin=[]  KbOutMax=[]  KtOutMin=[]  KtOutMax=[]  IntegratorOutMin=[]  IntegratorOutMax=[]  FilterOutMin=[]  FilterOutMax=[]  SumI1OutMin=[]  SumI1OutMax=[]  SumI2OutMin=[]  SumI2OutMax=[]  SumI3OutMin=[]  SumI3OutMax=[]  SumI4OutMin=[]  SumI4OutMax=[]  SumDOutMin=[]  SumDOutMax=[]  DifferentiatorOutMin=[]  DifferentiatorOutMax=[]  FilterDiffOutCoefMin=[]  FilterDiffOutCoefMax=[]  ReciprocalOutMin=[]  ReciprocalOutMax=[]  SumDenOutMin=[]  SumDenOutMax=[]  SumNumOutMin=[]  SumNumOutMax=[]  DivideOutMin=[]  DivideOutMax=[]  UdiffTsProdOutMin=[]  UdiffTsProdOutMax=[]  NTsProdOutMin=[]  NTsProdOutMax=[]  UintegralTsProdOutMin=[]  UintegralTsProdOutMax=[]  UngainTsProdOutMin=[]  UngainTsProdOutMax=[]  IntegratorContinuousStateAttributes=''  IntegratorStateMustResolveToSignalObject=off  IntegratorRTWStateStorageClass=Auto  FilterContinuousStateAttributes=''  FilterStateMustResolveToSignalObject=off  FilterRTWStateStorageClass=Auto  ParallelPVariant=InternalParameters  IdealPVariant=Disabled  IVariant=InternalParameters  DVariant=Disabled  IntegratorVariant=Continuous  SatVariant=Disabled  AWVariant=Passthrough  PCopyVariant=Disabled  TRVariant=Disabled  FdbkBlocksVariant=Forward  IdealPFdbkVariant=Disabled  SatFdbkVariant=Disabled  DerivativeFilterVariant=Disabled  NVariant=Disabled  NCopyVariant=Disabled_SignalSpec  FilterICVariant=Disabled  IntegratorICVariant=InternalICs  ExternalResetVariant=Disabled  TRSumVariant=Passthrough  SumFdbkVariant=Disabled  SumVariant=Sum_PI  TsampFilterVariant=InternalTs  TsampNgainVariant=Passthrough  TsampIntegralVariant=Passthrough  ExternalSaturationOutDataTypeStr=Inherit: Same as second input
  PWM Generator (DC-DC) : spsPWMGeneratorDCDCLib/PWM Generator (DC-DC)  Fsw=5000  Ts=0
  PWM Generator (DC-DC)1 : spsPWMGeneratorDCDCLib/PWM Generator (DC-DC)  Fsw=5000  Ts=0
  Saturation : Saturate
  Saturation1 : Saturate
  Sum : Sum  Inputs=|+-
  Switch : Switch  Criteria=u2 > Threshold
  D_PWM : Outport
  wires:
  Saturation/1 -> [D]
  [D] -> PWM Generator (DC-DC)/1
  I_PV/1 -> MATLAB Function/2(Ipv)
  V_PV/1 -> MATLAB Function/1(Vpv)
  MATLAB Function/1(D) -> Saturation/1
  Sum/1 -> PID Controller/1
  V_DC/1 -> Sum/2
  Constant/1 -> Sum/1
  PID Controller/1 -> Saturation1/1
  Switch/1 -> D_PWM/1
  Saturation1/1 -> PWM Generator (DC-DC)1/1
  Compare To Constant/1 -> Switch/2
  SOC_B/1 -> Compare To Constant/1
  PWM Generator (DC-DC)/1 -> Switch/3
  PWM Generator (DC-DC)1/1 -> Switch/1

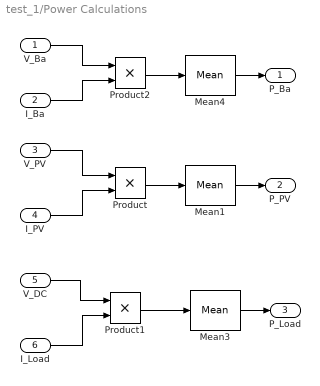
== system test_1/Power Calculations ==
  V_Ba : Inport
  I_Ba : Inport  Port=2
  V_PV : Inport  Port=3
  I_PV : Inport  Port=4
  V_DC : Inport  Port=5
  I_Load : Inport  Port=6
  Mean1 : spsMeanLib/Mean  Freq=60  Vinit=0  Ts=0
  Mean3 : spsMeanLib/Mean  Freq=60  Vinit=0  Ts=0
  Mean4 : spsMeanLib/Mean  Freq=60  Vinit=0  Ts=0
  Product : Product
  Product1 : Product
  Product2 : Product
  P_Ba : Outport
  P_PV : Outport  Port=2
  P_Load : Outport  Port=3
  wires:
  I_Ba/1 -> Product2/2
  V_Ba/1 -> Product2/1
  V_PV/1 -> Product/1
  I_PV/1 -> Product/2
  V_DC/1 -> Product1/1
  I_Load/1 -> Product1/2
  Mean4/1 -> P_Ba/1
  Product2/1 -> Mean4/1
  Mean1/1 -> P_PV/1
  Product/1 -> Mean1/1
  Mean3/1 -> P_Load/1
  Product1/1 -> Mean3/1

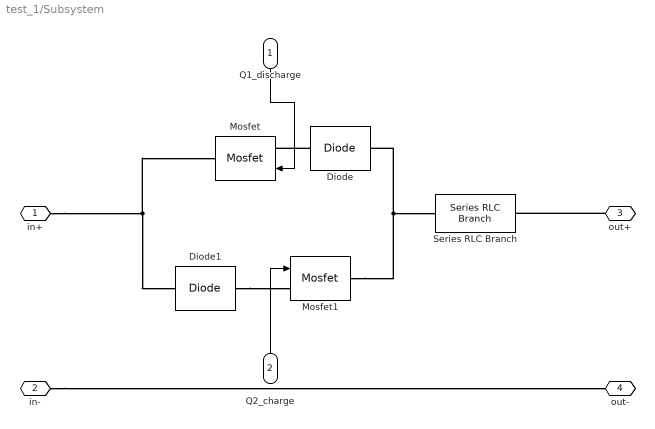
== system test_1/Subsystem ==
  Q1_discharge : Inport
  Q2_charge : Inport  Port=2
  Diode : spsDiodeLib/Diode  Ron=0.001  Lon=0  Vf=0.8  IC=0  UseSnubber=0  Rs=500  Cs=250e-9  Measurements=off
  Diode1 : spsDiodeLib/Diode  Ron=0.001  Lon=0  Vf=0.8  IC=0  UseSnubber=0  Rs=500  Cs=250e-9  Measurements=off
  Mosfet : spsMosfetLib/Mosfet  Ron=0.1  Lon=0  Rd=0.01  Vfd=0  IC=0  Rs=1e5  Cs=inf  Measurements=off
  Mosfet1 : spsMosfetLib/Mosfet  Ron=0.1  Lon=0  Rd=0.01  Vfd=0  IC=0  Rs=1e5  Cs=inf  Measurements=off
  Series RLC Branch : spsSeriesRLCBranchLib/Series RLC Branch  LConnTagsString=__new0  RConnTagsString=__new0  BranchType=RL  Resistance=0.05  Inductance=2.5e-3  SetiL0=off  InitialCurrent=0  Capacitance=1e-6  Setx0=off  InitialVoltage=0  Measurements=None
  in+ : PMIOPort  Side=Left
  in- : PMIOPort  Port=2  Side=Left
  out+ : PMIOPort  Port=3  Side=Right
  out- : PMIOPort  Port=4  Side=Right
  wires:
  Q2_charge/1 -> Mosfet1/1
  Q1_discharge/1 -> Mosfet/1
  connections:
  in-/RConn1 -- out-/RConn1
  out+/RConn1 -- Series RLC Branch/RConn1
  in+/RConn1 -- Diode1/RConn1 -- Mosfet/RConn1
  Diode/LConn1 -- Mosfet/LConn1
  Mosfet1/RConn1 -- Diode/RConn1 -- Series RLC Branch/LConn1
  Diode1/LConn1 -- Mosfet1/LConn1

== system test_1/Subsystem1 ==
  S_bt : Inport
  discharge_soc : Inport  Port=2
  charge_soc : Inport  Port=3
  NOT : Logic  Operator=NOT  IconShape=distinctive  AllPortsSameDT=off  OutDataTypeStr=boolean
  NOT1 : Logic  Operator=NOT  IconShape=distinctive  AllPortsSameDT=off  OutDataTypeStr=boolean
  Relational Operator : RelationalOperator  Operator=<=  OutDataTypeStr=boolean  RndMeth=Simplest
  Relational Operator1 : RelationalOperator  Operator===  OutDataTypeStr=boolean  RndMeth=Simplest
  Q1_discharge : Outport
  Q2_charge : Outport  Port=2
  wires:
  Relational Operator/1 -> NOT/1
  NOT/1 -> Q1_discharge/1
  discharge_soc/1 -> Relational Operator/2
  charge_soc/1 -> Relational Operator1/2
  NOT1/1 -> Q2_charge/1
  Relational Operator1/1 -> NOT1/1
  S_bt/1 -> Relational Operator1/1, Relational Operator/1

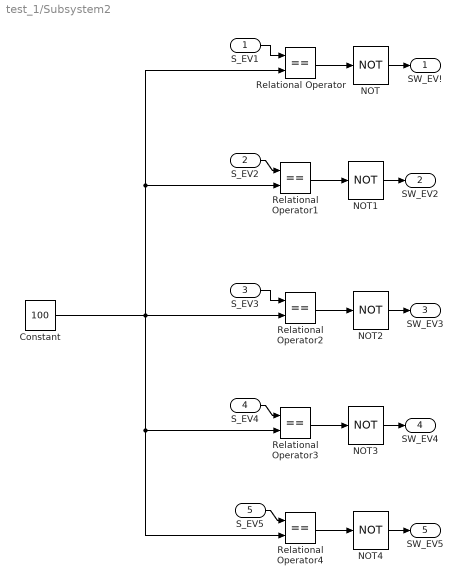
== system test_1/Subsystem2 ==
  S_EV1 : Inport
  S_EV2 : Inport  Port=2
  S_EV3 : Inport  Port=3
  S_EV4 : Inport  Port=4
  S_EV5 : Inport  Port=5
  Constant : Constant  Value=100
  NOT{,1..4} (5 alike) : Logic  Operator=NOT  IconShape=distinctive  AllPortsSameDT=off  OutDataTypeStr=boolean
  Relational Operator{,1..4} (5 alike) : RelationalOperator  Operator===  OutDataTypeStr=boolean  RndMeth=Simplest
  SW_EV! : Outport
  SW_EV2 : Outport  Port=2
  SW_EV3 : Outport  Port=3
  SW_EV4 : Outport  Port=4
  SW_EV5 : Outport  Port=5
  wires:
  Relational Operator1/1 -> NOT1/1
  S_EV1/1 -> Relational Operator/1
  S_EV2/1 -> Relational Operator1/1
  Relational Operator/1 -> NOT/1
  NOT1/1 -> SW_EV2/1
  NOT/1 -> SW_EV!/1
  NOT2/1 -> SW_EV3/1
  NOT3/1 -> SW_EV4/1
  Relational Operator2/1 -> NOT2/1
  S_EV4/1 -> Relational Operator3/1
  S_EV3/1 -> Relational Operator2/1
  Relational Operator3/1 -> NOT3/1
  Relational Operator4/1 -> NOT4/1
  S_EV5/1 -> Relational Operator4/1
  NOT4/1 -> SW_EV5/1
  Constant/1 -> Relational Operator1/2, Relational Operator/2, Relational Operator2/2, Relational Operator4/2, Relational Operator3/2

== matlab function test_1/MPPT PnO/MATLAB Function ==
  settings: updateMethod=DISCRETE  sampleTime=1e-4
  data: Vpv input; D output; Ipv input
function D = PandO(Vpv,Ipv)

persistent Dold Pold Vold


if isempty(Dold)
    Dold = 0.35;
    Vold = 17;
    Pold = 120;
end


deltaD = 0.001;

Ppv = Vpv*Ipv;

if (Ppv-Pold) ~= 0
    if (Ppv-Pold) > 0
        if (Vpv-Vold) > 0
            D = Dold - deltaD;
        else
            D = Dold + deltaD;
        end
    else
        if (Vpv-Vold) > 0
            D = Dold + deltaD;
        else
            D = Dold - deltaD;
        end        
    end
else
    D = Dold;
end

Dold = D;
Vold = Vpv;
Pold = Ppv;
